simulink model "Carla"  (R2019a)
settings: Solver=VariableStepAuto  StartTime=0.0  StopTime=inf  RelTol=1e-3
libraries: visionsinks x4
settings Model: Creator=darks  LastModifiedBy=darks

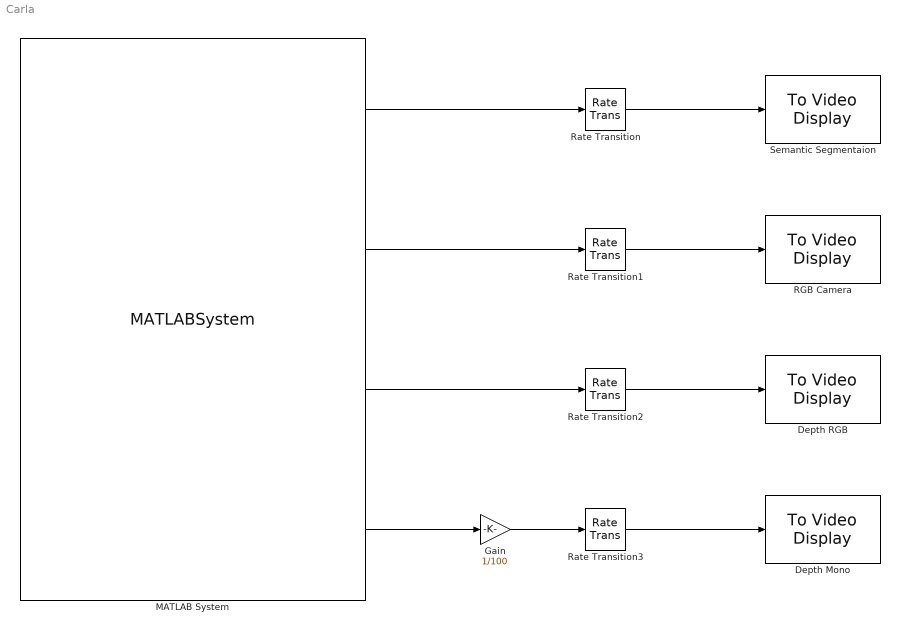
== system Carla ==
  Depth Mono : visionsinks/To Video Display  windowSizeMode=Normal  openAtMdlStart=on  fullScreen=off  videoWindowX=536805376  videoWindowY=536805376  saveWindowSize=off  videoWindowWidth=2147483647  videoWindowHeight=2147483647  inputColorFormat=RGB  inputType=Obsolete  imagePorts=One multidimensional signal  OutputDevice=On-screen video monitor  dataOrg=Column-major  isWindowOpen=off
      settings: SourceProductName=Computer Vision Toolbox
  Depth RGB : visionsinks/To Video Display  windowSizeMode=Normal  openAtMdlStart=on  fullScreen=off  videoWindowX=536805376  videoWindowY=536805376  saveWindowSize=off  videoWindowWidth=2147483647  videoWindowHeight=2147483647  inputColorFormat=RGB  inputType=Obsolete  imagePorts=One multidimensional signal  OutputDevice=On-screen video monitor  dataOrg=Column-major  isWindowOpen=off
      settings: SourceProductName=Computer Vision Toolbox
  Gain : Gain  Gain=1/100  OutDataTypeStr=Inherit: Same as input
  MATLAB System : MATLABSystem  System=CarlaEnvironment  SimulateUsing=Interpreted execution
      mask Type: CarlaEnvironment
      mask Display:
      | disp('CarlaEnvironment');
      | port_label('output',1,'SEMANTIC_SEGMENTATION_RGB');
      | port_label('output',2,'RGB');
      | port_label('output',3,'DEPTH_RBG');
      | port_label('output',4,'DEPTH');
  RGB Camera : visionsinks/To Video Display  windowSizeMode=Normal  openAtMdlStart=on  fullScreen=off  videoWindowX=536805376  videoWindowY=536805376  saveWindowSize=off  videoWindowWidth=2147483647  videoWindowHeight=2147483647  inputColorFormat=RGB  inputType=Obsolete  imagePorts=One multidimensional signal  OutputDevice=On-screen video monitor  dataOrg=Column-major  isWindowOpen=off
      settings: SourceProductName=Computer Vision Toolbox
  Rate Transition{,1..3} (4 alike) : RateTransition  OutPortSampleTime=.1
  Semantic Segmentaion : visionsinks/To Video Display  windowSizeMode=Normal  openAtMdlStart=on  fullScreen=off  videoWindowX=536805376  videoWindowY=536805376  saveWindowSize=off  videoWindowWidth=2147483647  videoWindowHeight=2147483647  inputColorFormat=RGB  inputType=Obsolete  imagePorts=One multidimensional signal  OutputDevice=On-screen video monitor  dataOrg=Column-major  isWindowOpen=off
      settings: SourceProductName=Computer Vision Toolbox
  wires:
  Rate Transition/1 -> Semantic Segmentaion/1
  MATLAB System/1 -> Rate Transition/1
  MATLAB System/2 -> Rate Transition1/1
  Rate Transition1/1 -> RGB Camera/1
  Rate Transition2/1 -> Depth RGB/1
  MATLAB System/3 -> Rate Transition2/1
  MATLAB System/4 -> Gain/1
  Gain/1 -> Rate Transition3/1
  Rate Transition3/1 -> Depth Mono/1
